simulink model "VDSE_2018b"  (R2018b)
settings: Solver=ode5  StartTime=0.0  StopTime=T_simulation  FixedStep=simulation_step_time  RelTol=1e-3
values from neighbouring files (symbols this model uses):
  A = 2    [vehicle_parameters_script.m]
  bump_height = 0    [vehicle_parameters_script.m]
  bump_length = 1    [vehicle_parameters_script.m]
  bump_time = 1    [vehicle_parameters_script.m]
  Bxf = 17.156    [BCD_Parameters.m]
  Bxr = 17.156    [BCD_Parameters.m]
  Byf = 12.71    [BCD_Parameters.m]
  Byr = 12.71    [BCD_Parameters.m]
  cd = 0.35    [vehicle_parameters_script.m]
  central_diff = 1    [vehicle_parameters_script.m]
  cF = 5000    [vehicle_parameters_script.m]
  clF = -0.15    [vehicle_parameters_script.m]
  clR = -0.20    (= -0.2)    [vehicle_parameters_script.m]
  cp_FA = 30    [vehicle_parameters_script.m]
  cp_RA = 13    [vehicle_parameters_script.m]
  cR = 5000    [vehicle_parameters_script.m]
  ctF = tireF.VERTICAL_DAMPING    [vehicle_parameters_script.m]
  ctR = tireR.VERTICAL_DAMPING    [vehicle_parameters_script.m]
  Cxf = 1.406    [BCD_Parameters.m]
  Cxr = 1.406    [BCD_Parameters.m]
  Cyf = 1.63    [BCD_Parameters.m]
  Cyr = 1.63    [BCD_Parameters.m]
  Dxf = 1.2    [BCD_Parameters.m]
  Dxr = 1.2    [BCD_Parameters.m]
  Dyf = 1.1    [BCD_Parameters.m]
  Dyr = 1.8    [BCD_Parameters.m]
  enableDriverControl = 0    [vehicle_parameters_script.m]
  enableLongDynamics = 1    [vehicle_parameters_script.m]
  enablePowertrain = 1    [vehicle_parameters_script.m]
  front_dr = 3.8    [vehicle_parameters_script.m]
  g = 9.806    [vehicle_parameters_script.m]
  Gear_numbers = [1 2 3 4 5 6]    [vehicle_parameters_script.m]
  GR = [2.9 1.8 1.3 1 0.85 0.75]    [vehicle_parameters_script.m]
  hcog = 0.5    [vehicle_parameters_script.m]
  hpc = 0.0    (= 0)    [vehicle_parameters_script.m]
  hrcF = 0.3    [vehicle_parameters_script.m]
  hrcg = (hrcF*lR+hrcR*lF)/(lF+lR)    (= 0.25108)    [vehicle_parameters_script.m]
  hrcR = 0.2    [vehicle_parameters_script.m]
  huFcog = 0.32    [vehicle_parameters_script.m]
  huRcog = 0.32    [vehicle_parameters_script.m]
  initial_gear = 1    [vehicle_parameters_script.m]
  JwF = 2.45    [vehicle_parameters_script.m]
  JwR = 2.45    [vehicle_parameters_script.m]
  Jx = 430    [vehicle_parameters_script.m]
  Jy = 1309    [vehicle_parameters_script.m]
  Jz = 1461    [vehicle_parameters_script.m]
  kF = 40000    [vehicle_parameters_script.m]
  kR = 35000    [vehicle_parameters_script.m]
  kRF = 0    [vehicle_parameters_script.m]
  kRR = 0    [vehicle_parameters_script.m]
  ktF = tireF.VERTICAL_STIFFNESS    [vehicle_parameters_script.m]
  ktR = tireR.VERTICAL_STIFFNESS    [vehicle_parameters_script.m]
  lF = 1.223    [vehicle_parameters_script.m]
  lR = l-lF    (= 1.277)    [vehicle_parameters_script.m]
  m = 1310    [vehicle_parameters_script.m]
  max_pressure = 1000    [vehicle_parameters_script.m]
  maxrpm = 4000    [vehicle_parameters_script.m]
  mF = 45    [vehicle_parameters_script.m]
  minrpm = 1500    [vehicle_parameters_script.m]
  mR = 50    [vehicle_parameters_script.m]
  output_samping_time = 0.001    [vehicle_parameters_script.m]
  phi0 = 0    [vehicle_parameters_script.m]
  phi_dot0 = 0    [vehicle_parameters_script.m]
  psi0 = 0    [vehicle_parameters_script.m]
  psi_dot0 = 0    [vehicle_parameters_script.m]
  rear_dr = 3.8    [vehicle_parameters_script.m]
  requested_speed = 100/3.6    (= 27.7777777778)    [vehicle_parameters_script.m]
  rF = tireF.UNLOADED_RADIUS    [vehicle_parameters_script.m]
  rho = 1.2    [vehicle_parameters_script.m]
  RPMME = Engine(:,1)    [vehicle_parameters_script.m]
  rR = tireR.UNLOADED_RADIUS    [vehicle_parameters_script.m]
  steer_ratio = 13.25    [vehicle_parameters_script.m]
  TFL = 0    [vehicle_parameters_script.m]
  TFR = 0    [vehicle_parameters_script.m]
  theta0 = 0    [vehicle_parameters_script.m]
  theta_dot0 = 0    [vehicle_parameters_script.m]
  TorqueME = []    [vehicle_parameters_script.m]
  TRL = 0    [vehicle_parameters_script.m]
  TRR = 0    [vehicle_parameters_script.m]
  Vx0 = 100/3.6    (= 27.7777777778)    [vehicle_parameters_script.m]
  Vy0 = 0    [vehicle_parameters_script.m]
  Vz0 = 0    [vehicle_parameters_script.m]
  wF = 1.578    [vehicle_parameters_script.m]
  wR = 1.544    [vehicle_parameters_script.m]
  x0 = 0    [vehicle_parameters_script.m]
  xcog_overall = (2*mR*xR+2*xF*mF+m*xs)/(m+2*mF+2*mR)    (= 1.23475333333)    [vehicle_parameters_script.m]
  y0 = 0    [vehicle_parameters_script.m]
  z0 = 0    [vehicle_parameters_script.m]
  zFL0 = 0    [vehicle_parameters_script.m]
  zFL_dot0 = 0    [vehicle_parameters_script.m]
  zFR0 = 0    [vehicle_parameters_script.m]
  zFR_dot0 = 0    [vehicle_parameters_script.m]
  zRL0 = 0    [vehicle_parameters_script.m]
  zRL_dot0 = 0    [vehicle_parameters_script.m]
  zRR0 = 0    [vehicle_parameters_script.m]
  zRR_dot0 = 0    [vehicle_parameters_script.m]
undefined symbols (not defined in the file or in its folder): exf, exr, eyf, eyr, FNOMINf, FNOMINr, PCX1f, PCX1r, PCY1f, PCY1r, PDX1f, PDX1r, PDX2f, PDX2r, PDY1f, PDY1r, PDY2f, PDY2r, PDY3f, PDY3r, PEX1f, PEX1r, PEX2f, PEX2r, PEX3f, PEX3r, PEX4f, PEX4r, PEY1f, PEY1r, PEY2f, PEY2r, PEY3f, PEY3r, PEY4f, PEY4r, PHX1f, PHX1r, PHX2f, PHX2r, PHY1f, PHY1r, PHY2f, PHY2r, PHY3f, PHY3r, PKX1f, PKX1r, PKX2f, PKX2r, PKX3f, PKX3r, PKY1f, PKY1r, PKY2f, PKY2r, PKY3f, PKY3r, PVX1f, PVX1r ... (+122)
libraries: simulink x7, mfeval_LIB x4
(part 1 of 6)
settings Model: Creator=Christos  LastModifiedBy=Christos

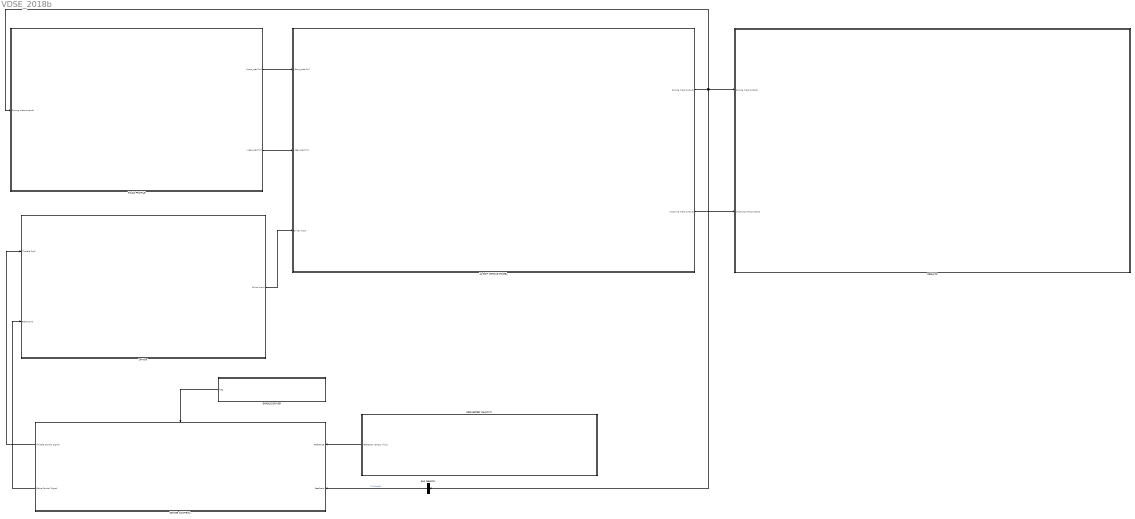
== system VDSE_2018b ==
  14-DOF VEHICLE MODEL : Subsystem
  Bus Selector : BusSelector  OutputSignals=Longitudinal Dynamics.Vx [m/s]
  DRIVER : Subsystem
  DRIVER CONTROL : Subsystem  TreatAsAtomicUnit=on
  "ENABLE DRIVER " : Subsystem
  REQUESTED VELOCITY : Subsystem
  RESULTS : Subsystem
  ROAD PROFILE : Subsystem
  wires:
  14-DOF VEHICLE MODEL/2(Unsprung mass outputs) -> RESULTS/2(Unsprung mass outputs)
  ROAD PROFILE/2(yrear_road [m]) -> 14-DOF VEHICLE MODEL/2(yrear_road [m])
  Bus Selector/1 -> DRIVER CONTROL/2(Feedback)  "<Vx [m/s]>"
  ROAD PROFILE/1(yfront_road [m]) -> 14-DOF VEHICLE MODEL/1(yfront_road [m])
  DRIVER/1(Driver Input) -> 14-DOF VEHICLE MODEL/3(Driver Input)
  DRIVER CONTROL/2(Brake Control Signal) -> DRIVER/2(Brake Cmd)
  14-DOF VEHICLE MODEL/1(Sprung mass outputs) -> Bus Selector/1, RESULTS/1(Sprung mass outputs), ROAD PROFILE/1(Sprung mass outputs)
  DRIVER CONTROL/1(Throttle Control Signal) -> DRIVER/1(Throttle Cmd)
  REQUESTED VELOCITY/1(reference velocity [m/s]) -> DRIVER CONTROL/1(Reference)
  "ENABLE DRIVER "/1(flag) -> DRIVER CONTROL/Enable

== system VDSE_2018b/14-DOF VEHICLE MODEL ==
  yfront_road [m] : Inport
  yrear_road [m] : Inport  Port=2
  Driver Input : Inport  Port=3
  Driver Input1 : InportShadow  Port=3
  EQUATIONS OF MOTION FOR CHASSIS : Subsystem
  POWERTRAIN AND BRAKES : Subsystem
  SUSPENSION : Subsystem
  WHEEL ASSEMBLY : Subsystem  Variant=on
  Sprung mass outputs : Outport
  Unsprung mass outputs : Outport  Port=2
  wires:
  EQUATIONS OF MOTION FOR CHASSIS/1(Sprung mass outputs) -> Sprung mass outputs/1, SUSPENSION/3(sprung mass outputs), WHEEL ASSEMBLY/2(sprung mass outputs)  "Sprung mass outputs"
  yfront_road [m]/1 -> SUSPENSION/1(yfront_road [m])
  yrear_road [m]/1 -> SUSPENSION/2(yrear_road [m])
  WHEEL ASSEMBLY/1(Tyre Forces and Moments) -> EQUATIONS OF MOTION FOR CHASSIS/2(Tyre Forces and Moments)
  SUSPENSION/1(" Unsprung masses output") -> WHEEL ASSEMBLY/3(unsprung masses outputs), EQUATIONS OF MOTION FOR CHASSIS/3(unsprung masses outputs), Unsprung mass outputs/1  "unsprung masses outputs"
  Driver Input/1 -> EQUATIONS OF MOTION FOR CHASSIS/1(Steer Input [rad]), WHEEL ASSEMBLY/1(steer input [rad])
  WHEEL ASSEMBLY/2(Wheel Speeds [rad/s]) -> POWERTRAIN AND BRAKES/1(Wheels speed [rad/s])
  Driver Input1/1 -> POWERTRAIN AND BRAKES/2(Driver)
  POWERTRAIN AND BRAKES/1(Torques [Nm]) -> [Torques]
  [Torques] -> WHEEL ASSEMBLY/4(Torques [Nm])

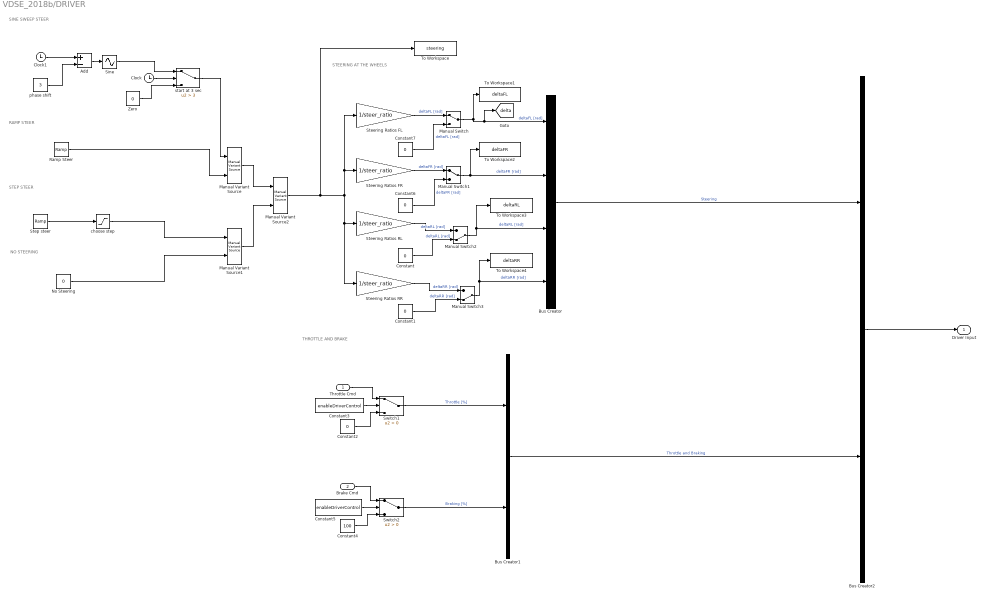
== system VDSE_2018b/DRIVER ==
  note: THROTTLE AND BRAKE
  note: STEERING AT THE WHEELS
  note: NO STEERING
  note: STEP STEER
  note: RAMP STEER
  note: SINE SWEEP STEER
  Throttle Cmd : Inport
  Brake Cmd : Inport  Port=2
  Add : Sum  Inputs=+-
  Bus Creator : BusCreator  Inputs=4
  Bus Creator1 : BusCreator  Inputs=2
  Bus Creator2 : BusCreator  Inputs=2
  Clock : Clock
  Clock1 : Clock
  Constant{,1..2,6..7} (5 alike) : Constant  Value=0
  Constant3 : Constant  Value=enableDriverControl
  Constant4 : Constant  Value=100
  Constant5 : Constant  Value=enableDriverControl
  Manual Variant Source : simulink/Signal Routing/Manual Variant Source  NumChoices=2  LabelModeActiveChoice=V_2
      settings: SourceProductName=Simulink
  Manual Variant Source1 : simulink/Signal Routing/Manual Variant Source  NumChoices=2  LabelModeActiveChoice=V_2
      settings: SourceProductName=Simulink
  Manual Variant Source2 : simulink/Signal Routing/Manual Variant Source  NumChoices=2  LabelModeActiveChoice=V_1
      settings: SourceProductName=Simulink
  Manual Switch : ManualSwitch
  Manual Switch1 : ManualSwitch
  Manual Switch2 : ManualSwitch  CurrentSetting=0
  Manual Switch3 : ManualSwitch  CurrentSetting=0
  No Steering : Constant  Value=0
  Ramp Steer : simulink/Sources/Ramp  slope=10*pi/180  start=1  InitialOutput=0
  Sine : Sin  TimeSource=Use external signal  Amplitude=30*pi/180  SampleTime=0
  Steering Ratios FL : Gain  Gain=1/steer_ratio
  Steering Ratios FR : Gain  Gain=1/steer_ratio
  Steering Ratios RL : Gain  Gain=1/steer_ratio
  Steering Ratios RR : Gain  Gain=1/steer_ratio
  Step steer : simulink/Sources/Ramp  slope=1400*pi/180  start=15  InitialOutput=0
  Switch1 : Switch  Criteria=u2 > Threshold
  Switch2 : Switch  Criteria=u2 > Threshold
  To Workspace : ToWorkspace  VariableName=steering  SaveFormat=Timeseries  SampleTime=output_samping_time
  To Workspace1 : ToWorkspace  VariableName=deltaFL  SaveFormat=Timeseries  SampleTime=output_samping_time
  To Workspace2 : ToWorkspace  VariableName=deltaFR  SaveFormat=Timeseries  SampleTime=output_samping_time
  To Workspace3 : ToWorkspace  VariableName=deltaRL  SaveFormat=Timeseries  SampleTime=output_samping_time
  To Workspace4 : ToWorkspace  VariableName=deltaRR  SaveFormat=Timeseries  SampleTime=output_samping_time
  Zero : Constant  Value=0  OutDataTypeStr=Inherit: Inherit via back propagation
  "choose step " : Saturate  UpperLimit=700*pi/180  LowerLimit=0
  "phase shift " : Constant  Value=3
  start at 3 sec : Switch  Criteria=u2 > Threshold  Threshold=3
  Driver Input : Outport
  tag scope: delta=global
  wires:
  Zero/1 -> start at 3 sec/3
  Manual Switch3/1 -> To Workspace4/1, Bus Creator/4  "deltaRR [rad]"
  "phase shift "/1 -> Add/2
  Add/1 -> Sine/1
  Clock1/1 -> Add/1
  Clock/1 -> start at 3 sec/2
  start at 3 sec/1 -> Manual Variant Source/1
  "choose step "/1 -> Manual Variant Source1/1
  Manual Variant Source/1 -> Manual Variant Source2/1
  Sine/1 -> start at 3 sec/1
  No Steering/1 -> Manual Variant Source1/2
  Manual Variant Source1/1 -> Manual Variant Source2/2
  Manual Switch/1 -> [delta], Bus Creator/1, To Workspace1/1  "deltaFL [rad]"
  Manual Variant Source2/1 -> To Workspace/1, Steering Ratios FL/1, Steering Ratios FR/1, Steering Ratios RL/1, Steering Ratios RR/1
  Step steer/1 -> "choose step "/1
  Ramp Steer/1 -> Manual Variant Source/2
  Manual Switch2/1 -> To Workspace3/1, Bus Creator/3  "deltaRL [rad]"
  Constant2/1 -> Switch1/3
  Bus Creator2/1 -> Driver Input/1
  Bus Creator/1 -> Bus Creator2/1  "Steering"
  Bus Creator1/1 -> Bus Creator2/2  "Throttle and Braking"
  Throttle Cmd/1 -> Switch1/1
  Constant3/1 -> Switch1/2
  Constant1/1 -> Manual Switch3/2  "deltaRR [rad]"
  Constant/1 -> Manual Switch2/2  "deltaRL [rad]"
  Steering Ratios RL/1 -> Manual Switch2/1  "deltaRL [rad]"
  Steering Ratios FL/1 -> Manual Switch/1  "deltaFL [rad]"
  Manual Switch1/1 -> To Workspace2/1, Bus Creator/2  "deltaFR [rad]"
  Steering Ratios FR/1 -> Manual Switch1/1  "deltaFR [rad]"
  Brake Cmd/1 -> Switch2/1
  Constant5/1 -> Switch2/2
  Constant4/1 -> Switch2/3
  Switch2/1 -> Bus Creator1/2  "Braking [%]"
  Constant6/1 -> Manual Switch1/2  "deltaFR [rad]"
  Constant7/1 -> Manual Switch/2  "deltaFL [rad]"
  Switch1/1 -> Bus Creator1/1  "Throttle [%]"
  Steering Ratios RR/1 -> Manual Switch3/1  "deltaRR [rad]"

== system VDSE_2018b/DRIVER CONTROL ==
  Reference : Inport
  Feedback : Inport  Port=2
  Enable : EnablePort
  Abs : Abs
  Add : Sum  Inputs=+-
  Driver : simulink/Continuous/PID Controller  Controller=PID  Form=Parallel  TimeDomain=Continuous-time  SampleTime=-1  IntegratorMethod=Forward Euler  FilterMethod=Forward Euler  ControllerParametersSource=internal  P=200  I=0  D=50  UseFilter=on  N=10  TunerSelectOption=Transfer Function Based (PID Tuner App)  InitialConditionSource=internal  InitialConditionForIntegrator=0  InitialConditionForFilter=0  DifferentiatorICPrevScaledInput=0  ExternalReset=none  TrackingMode=off  Kt=1  LimitOutput=off  UpperSaturationLimit=inf  LowerSaturationLimit=-inf  LinearizeAsGain=on  AntiWindupMode=none  Kb=1  POutMin=[]  POutMax=[]  IOutMin=[]  IOutMax=[]  DOutMin=[]  DOutMax=[]  NOutMin=[]  NOutMax=[]  SumOutMin=[]  SumOutMax=[]  SaturationOutMin=[]  SaturationOutMax=[]  PParamMin=[]  PParamMax=[]  IParamMin=[]  IParamMax=[]  DParamMin=[]  DParamMax=[]  NParamMin=[]  NParamMax=[]  KbParamMin=[]  KbParamMax=[]  KtParamMin=[]  KtParamMax=[]  KbOutMin=[]  KbOutMax=[]  KtOutMin=[]  KtOutMax=[]  IntegratorOutMin=[]  IntegratorOutMax=[]  FilterOutMin=[]  FilterOutMax=[]  SumI1OutMin=[]  SumI1OutMax=[]  SumI2OutMin=[]  SumI2OutMax=[]  SumI3OutMin=[]  SumI3OutMax=[]  SumI4OutMin=[]  SumI4OutMax=[]  SumDOutMin=[]  SumDOutMax=[]  DifferentiatorOutMin=[]  DifferentiatorOutMax=[]  FilterDiffOutCoefMin=[]  FilterDiffOutCoefMax=[]  ReciprocalOutMin=[]  ReciprocalOutMax=[]  SumDenOutMin=[]  SumDenOutMax=[]  SumNumOutMin=[]  SumNumOutMax=[]  DivideOutMin=[]  DivideOutMax=[]  IntegratorContinuousStateAttributes=''  IntegratorStateMustResolveToSignalObject=off  IntegratorRTWStateStorageClass=Auto  FilterContinuousStateAttributes=''  FilterStateMustResolveToSignalObject=off  FilterRTWStateStorageClass=Auto  ParallelPVariant=InternalParameters  IdealPVariant=Disabled  IVariant=InternalParameters  DVariant=InternalParameters  IntegratorVariant=Continuous  SatVariant=Disabled  AWVariant=Passthrough  PCopyVariant=Disabled  TRVariant=Disabled  FdbkBlocksVariant=Forward  IdealPFdbkVariant=Disabled  SatFdbkVariant=Disabled  DerivativeFilterVariant=ContFilter  NVariant=InternalParameters  NCopyVariant=Disabled  FilterICVariant=InternalICsFilter  IntegratorICVariant=InternalICs  ExternalResetVariant=Disabled  TRSumVariant=Passthrough  SumFdbkVariant=Disabled  SumVariant=Sum_PID
  MATLAB Function : MATLAB Function  TreatAsAtomicUnit=on
  Saturation : Saturate  UpperLimit=100  LowerLimit=0
  Saturation1 : Saturate  UpperLimit=0  LowerLimit=-100
  Scope : Scope  NumInputPorts=2
  Scope1 : Scope
  Throttle Control Signal : Outport
  Brake Control Signal : Outport  Port=2
  wires:
  Reference/1 -> Add/1
  Add/1 -> Scope1/1, Driver/1  "Error"
  Driver/1 -> Saturation/1, Saturation1/1
  Saturation/1 -> Scope/1, Throttle Control Signal/1  "Throttle Command [%]"
  Saturation1/1 -> Scope/2, MATLAB Function/1(brake)  "Brake Command [%]"
  MATLAB Function/1(Brake_Cmd) -> Abs/1
  Feedback/1 -> MATLAB Function/2(Vx), Add/2
  Abs/1 -> Brake Control Signal/1

== system VDSE_2018b/ENABLE DRIVER  ==
  Constant1 : Constant  Value=enableDriverControl
  flag : Outport
  wires:
  Constant1/1 -> flag/1

== system VDSE_2018b/REQUESTED VELOCITY ==
  note: REQUESTED VELOCITY
  Constant : Constant  Value=requested_speed
  Manual Switch : ManualSwitch
  Sine Wave : Sin  Amplitude=10/3.6  Bias=90/3.6  Frequency=0.1  SampleTime=0
  reference velocity [m/s] : Outport
  tag scope: ref_vel=global
  wires:
  Manual Switch/1 -> reference velocity [m/s]/1, [ref_vel]  "reference velocity [m/s]"
  Sine Wave/1 -> Manual Switch/2
  Constant/1 -> Manual Switch/1

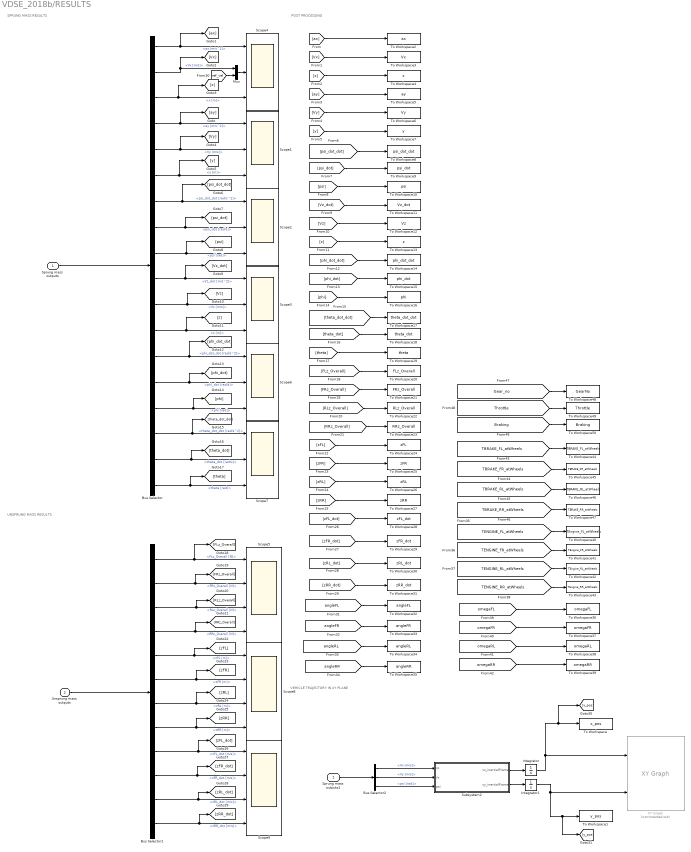
== system VDSE_2018b/RESULTS ==
  note: POST PROCESSING
  note: VEHICLE TRAJECTORY IN XY PLANE
  note: UNSPRUNG MASS RESULTS
  note: SPRUNG MASS RESULTS
  Sprung mass outputs : Inport
  Unsprung mass outputs : Inport  Port=2
  Bus Selector : BusSelector  OutputSignals=Longitudinal Dynamics.ax [m/s^2],Longitudinal Dynamics.Vx [m/s],Longitudinal Dynamics.x [m],Lateral Dynamics.ay [m/s^2],Lateral Dynamics.Vy [m/s],Lateral Dynamics.y [m],Yaw dynamics.psi_dot_dot [rad/s^2],Yaw dynamics.psi_dot [rad/s],Yaw dynamics.psi [rad],Vertical Dynamics.Vz_dot [m/s^2],Vertical Dynamics.Vz [m/s],Vertical Dynamics.z [m],Roll Dynamics.phi_dot_dot [rad/s^2],Roll Dynamics.phi_dot [rad/s],Roll Dynamics.phi [rad],Pitch Dynamics.theta_dot_dot [rad/s^2],Pitch Dynamics.theta_dot [rad/s],Pitch Dynamics.theta [rad]
  Bus Selector1 : BusSelector  OutputSignals=Unsprung masses z Forces [N].FLz_Overall [N],Unsprung masses z Forces [N].FRz_Overall [N],Unsprung masses z Forces [N].RLz_Overall [N],Unsprung masses z Forces [N].RRz_Overall [N],Unsprung masses z displacement [m].zFL [m],Unsprung masses z displacement [m].zFR [m],Unsprung masses z displacement [m].zRL [m],Unsprung masses z displacement [m].zRR [m],Unsprung masses z Velocities [m/s].zFL_dot [m/s],Unsprung masses z Velocities [m/s].zFR_dot [m/s],Unsprung masses z Velocities [m/s].zRL_dot [m/s],Unsprung masses z Velocities [m/s].zRR_dot [m/s]
  Bus Selector2 : BusSelector  OutputSignals=Longitudinal Dynamics.Vx [m/s],Lateral Dynamics.Vy [m/s],Yaw dynamics.psi [rad]
  Integrator : Integrator
  Integrator1 : Integrator
  Mux : Mux  Inputs=2
  Scope{1..4,6..7} (6 alike) : Scope  NumInputPorts=3
  Scope5 : Scope  NumInputPorts=4
  Scope8 : Scope  NumInputPorts=4
  Scope9 : Scope  NumInputPorts=4
  Sprung mass outputs1 : InportShadow
  Subsystem2 : Subsystem
  To Workspace : ToWorkspace  VariableName=x_pos  SaveFormat=Timeseries  SampleTime=output_samping_time
  To Workspace1 : ToWorkspace  VariableName=y_pos  SaveFormat=Timeseries  SampleTime=output_samping_time
  To Workspace10 : ToWorkspace  VariableName=psi  SaveFormat=Timeseries  SampleTime=output_samping_time
  To Workspace11 : ToWorkspace  VariableName=Vz_dot  SaveFormat=Timeseries  SampleTime=output_samping_time
  To Workspace12 : ToWorkspace  VariableName=Vz  SaveFormat=Timeseries  SampleTime=output_samping_time
  To Workspace13 : ToWorkspace  VariableName=z  SaveFormat=Timeseries  SampleTime=output_samping_time
  To Workspace14 : ToWorkspace  VariableName=phi_dot_dot  SaveFormat=Timeseries  SampleTime=output_samping_time
  To Workspace15 : ToWorkspace  VariableName=phi_dot  SaveFormat=Timeseries  SampleTime=output_samping_time
  To Workspace16 : ToWorkspace  VariableName=phi  SaveFormat=Timeseries  SampleTime=output_samping_time
  To Workspace17 : ToWorkspace  VariableName=theta_dot_dot  SaveFormat=Timeseries  SampleTime=output_samping_time
  To Workspace18 : ToWorkspace  VariableName=theta_dot  SaveFormat=Timeseries  SampleTime=output_samping_time
  To Workspace19 : ToWorkspace  VariableName=theta  SaveFormat=Timeseries  SampleTime=output_samping_time
  To Workspace2 : ToWorkspace  VariableName=ax  SaveFormat=Timeseries  SampleTime=output_samping_time
  To Workspace20 : ToWorkspace  VariableName=FLz_Overall  SaveFormat=Timeseries  SampleTime=output_samping_time
  To Workspace21 : ToWorkspace  VariableName=FRz_Overall  SaveFormat=Timeseries  SampleTime=output_samping_time
  To Workspace22 : ToWorkspace  VariableName=RLz_Overall  SaveFormat=Timeseries  SampleTime=output_samping_time
  To Workspace23 : ToWorkspace  VariableName=RRz_Overall  SaveFormat=Timeseries  SampleTime=output_samping_time
  To Workspace24 : ToWorkspace  VariableName=zFL  SaveFormat=Timeseries  SampleTime=output_samping_time
  To Workspace25 : ToWorkspace  VariableName=zFR  SaveFormat=Timeseries  SampleTime=output_samping_time
  To Workspace26 : ToWorkspace  VariableName=zRL  SaveFormat=Timeseries  SampleTime=output_samping_time
  To Workspace27 : ToWorkspace  VariableName=zRR  SaveFormat=Timeseries  SampleTime=output_samping_time
  To Workspace28 : ToWorkspace  VariableName=zFL_dot  SaveFormat=Timeseries  SampleTime=output_samping_time
  To Workspace29 : ToWorkspace  VariableName=zFR_dot  SaveFormat=Timeseries  SampleTime=output_samping_time
  To Workspace3 : ToWorkspace  VariableName=Vx  SaveFormat=Timeseries  SampleTime=output_samping_time
  To Workspace30 : ToWorkspace  VariableName=zRL_dot  SaveFormat=Timeseries  SampleTime=output_samping_time
  To Workspace31 : ToWorkspace  VariableName=zRR_dot  SaveFormat=Timeseries  SampleTime=output_samping_time
  To Workspace32 : ToWorkspace  VariableName=angleFL  SaveFormat=Timeseries  SampleTime=output_samping_time
  To Workspace33 : ToWorkspace  VariableName=angleFR  SaveFormat=Timeseries  SampleTime=output_samping_time
  To Workspace34 : ToWorkspace  VariableName=angleRL  SaveFormat=Timeseries  SampleTime=output_samping_time
  To Workspace35 : ToWorkspace  VariableName=angleRR  SaveFormat=Timeseries  SampleTime=output_samping_time
  To Workspace36 : ToWorkspace  VariableName=omegaFL  SaveFormat=Timeseries  SampleTime=output_samping_time
  To Workspace37 : ToWorkspace  VariableName=omegaFR  SaveFormat=Timeseries  SampleTime=output_samping_time
  To Workspace38 : ToWorkspace  VariableName=omegaRL  SaveFormat=Timeseries  SampleTime=output_samping_time
  To Workspace39 : ToWorkspace  VariableName=omegaRR  SaveFormat=Timeseries  SampleTime=output_samping_time
  To Workspace4 : ToWorkspace  VariableName=x  SaveFormat=Timeseries  SampleTime=output_samping_time
  To Workspace40 : ToWorkspace  VariableName=TEngine_FL_atWheels  SaveFormat=Timeseries  SampleTime=output_samping_time
  To Workspace41 : ToWorkspace  VariableName=TEngine_FR_atWheels  SaveFormat=Timeseries  SampleTime=output_samping_time
  To Workspace42 : ToWorkspace  VariableName=TEngine_RL_atWheels  SaveFormat=Timeseries  SampleTime=output_samping_time
  To Workspace43 : ToWorkspace  VariableName=TEngine_RR_atWheels  SaveFormat=Timeseries  SampleTime=output_samping_time
  To Workspace44 : ToWorkspace  VariableName=TBRAKE_FL_atWheels  SaveFormat=Timeseries  SampleTime=output_samping_time
  To Workspace45 : ToWorkspace  VariableName=TBRAKE_FR_atWheels  SaveFormat=Timeseries  SampleTime=output_samping_time
  To Workspace46 : ToWorkspace  VariableName=TBRAKE_RL_atWheels  SaveFormat=Timeseries  SampleTime=output_samping_time
  To Workspace47 : ToWorkspace  VariableName=TBRAKE_RR_atWheels  SaveFormat=Timeseries  SampleTime=output_samping_time
  To Workspace48 : ToWorkspace  VariableName=GearNo  SaveFormat=Timeseries  SampleTime=output_samping_time
  To Workspace49 : ToWorkspace  VariableName=Throttle  SaveFormat=Timeseries  SampleTime=output_samping_time
  To Workspace5 : ToWorkspace  VariableName=ay  SaveFormat=Timeseries  SampleTime=output_samping_time
  To Workspace50 : ToWorkspace  VariableName=Braking  SaveFormat=Timeseries  SampleTime=output_samping_time
  To Workspace6 : ToWorkspace  VariableName=Vy  SaveFormat=Timeseries  SampleTime=output_samping_time
  To Workspace7 : ToWorkspace  VariableName=y  SaveFormat=Timeseries  SampleTime=output_samping_time
  To Workspace8 : ToWorkspace  VariableName=psi_dot_dot  SaveFormat=Timeseries  SampleTime=output_samping_time
  To Workspace9 : ToWorkspace  VariableName=psi_dot  SaveFormat=Timeseries  SampleTime=output_samping_time
  XY Graph : simulink/Sinks/XY Graph  Commented=on  xmin=-2500  xmax=1500  ymin=-2500  ymax=1500  st=-1
  wires:
  Integrator1/1 -> [y_pos], To Workspace1/1, XY Graph/2
  Integrator/1 -> [x_pos], To Workspace/1, XY Graph/1
  Subsystem2/1(vx_inertialFrame) -> Integrator/1
  Subsystem2/2(vy_inertialFrame) -> Integrator1/1
  Sprung mass outputs/1 -> Bus Selector/1
  Unsprung mass outputs/1 -> Bus Selector1/1
  Bus Selector/1 -> [ax], Scope4/1  "<ax [m/s^2]>"
  Bus Selector/2 -> Mux/1, [Vx]  "<Vx [m/s]>"
  Bus Selector/3 -> [x], Scope4/3  "<x [m]>"
  Bus Selector/4 -> [ay], Scope1/1  "<ay [m/s^2]>"
  Bus Selector/5 -> [Vy], Scope1/2  "<Vy [m/s]>"
  Bus Selector/6 -> [y], Scope1/3  "<y [m]>"
  Bus Selector/7 -> [psi_dot_dot], Scope2/1  "<psi_dot_dot [rad/s^2]>"
  Bus Selector/8 -> [psi_dot], Scope2/2  "<psi_dot [rad/s]>"
  Bus Selector/9 -> [psi], Scope2/3  "<psi [rad]>"
  Bus Selector/10 -> [Vz_dot], Scope3/1  "<Vz_dot [m/s^2]>"
  Bus Selector/11 -> [Vz], Scope3/2  "<Vz [m/s]>"
  Bus Selector/12 -> [z], Scope3/3  "<z [m]>"
  Bus Selector/13 -> [phi_dot_dot], Scope6/1  "<phi_dot_dot [rad/s^2]>"
  Bus Selector/14 -> [phi_dot], Scope6/2  "<phi_dot [rad/s]>"
  Bus Selector/15 -> [phi], Scope6/3  "<phi [rad]>"
  Bus Selector/16 -> [theta_dot_dot], Scope7/1  "<theta_dot_dot [rad/s^2]>"
  Bus Selector/17 -> [theta_dot], Scope7/2  "<theta_dot [rad/s]>"
  Bus Selector/18 -> [theta], Scope7/3  "<theta [rad]>"
  Bus Selector1/1 -> [FLz_Overall], Scope5/1  "<FLz_Overall [N]>"
  Bus Selector1/2 -> [FRz_Overall], Scope5/2  "<FRz_Overall [N]>"
  Bus Selector1/3 -> [RLz_Overall], Scope5/3  "<RLz_Overall [N]>"
  Bus Selector1/4 -> [RRz_Overall], Scope5/4  "<RRz_Overall [N]>"
  Bus Selector1/5 -> [zFL], Scope8/1  "<zFL [m]>"
  Bus Selector1/6 -> [zFR], Scope8/2  "<zFR [m]>"
  Bus Selector1/7 -> [zRL], Scope8/3  "<zRL [m]>"
  Bus Selector1/8 -> [zRR], Scope8/4  "<zRR [m]>"
  Bus Selector1/9 -> [zFL_dot], Scope9/1  "<zFL_dot [m/s]>"
  Bus Selector1/10 -> [zFR_dot], Scope9/2  "<zFR_dot [m/s]>"
  Bus Selector1/11 -> [zRL_dot], Scope9/3  "<zRL_dot [m/s]>"
  Bus Selector1/12 -> [zRR_dot], Scope9/4  "<zRR_dot [m/s]>"
  Sprung mass outputs1/1 -> Bus Selector2/1
  Bus Selector2/1 -> Subsystem2/1(vx)  "<Vx [m/s]>"
  Bus Selector2/2 -> Subsystem2/2(vy)  "<Vy [m/s]>"
  Bus Selector2/3 -> Subsystem2/3(psi)  "<psi [rad]>"
  [ax] -> To Workspace2/1
  [Vx] -> To Workspace3/1
  [x] -> To Workspace4/1
  [ay] -> To Workspace5/1
  [Vy] -> To Workspace6/1
  [y] -> To Workspace7/1
  [psi_dot_dot] -> To Workspace8/1
  [psi_dot] -> To Workspace9/1
  [psi] -> To Workspace10/1
  [Vz_dot] -> To Workspace11/1
  [Vz] -> To Workspace12/1
  [z] -> To Workspace13/1
  [phi_dot_dot] -> To Workspace14/1
  [phi_dot] -> To Workspace15/1
  [phi] -> To Workspace16/1
  [theta_dot_dot] -> To Workspace17/1
  [theta_dot] -> To Workspace18/1
  [theta] -> To Workspace19/1
  [FLz_Overall] -> To Workspace20/1
  [FRz_Overall] -> To Workspace21/1
  [RLz_Overall] -> To Workspace22/1
  [RRz_Overall] -> To Workspace23/1
  [zFL] -> To Workspace24/1
  [zFR] -> To Workspace25/1
  [zRL] -> To Workspace26/1
  [zRR] -> To Workspace27/1
  [zFL_dot] -> To Workspace28/1
  [zFR_dot] -> To Workspace29/1
  [zRL_dot] -> To Workspace30/1
  [zRR_dot] -> To Workspace31/1
  Mux/1 -> Scope4/2
  [ref_vel] -> Mux/2
  [angleFL] -> To Workspace32/1
  [angleFR] -> To Workspace33/1
  [angleRL] -> To Workspace34/1
  [angleRR] -> To Workspace35/1
  [omegaFL] -> To Workspace36/1
  [omegaFR] -> To Workspace37/1
  [omegaRL] -> To Workspace38/1
  [omegaRR] -> To Workspace39/1
  [TENGINE_FL_atWheels] -> To Workspace40/1
  [TENGINE_FR_atWheels] -> To Workspace41/1
  [TENGINE_RL_atWheels] -> To Workspace42/1
  [TENGINE_RR_atWheels] -> To Workspace43/1
  [TBRAKE_FL_atWheels] -> To Workspace44/1
  [TBRAKE_FR_atWheels] -> To Workspace45/1
  [TBRAKE_RL_atWheels] -> To Workspace46/1
  [TBRAKE_RR_atWheels] -> To Workspace47/1
  [Gear_no] -> To Workspace48/1
  [Throttle] -> To Workspace49/1
  [Braking] -> To Workspace50/1

== system VDSE_2018b/ROAD PROFILE ==
  note: GENERATION OF ROAD PROFILE
  Sprung mass outputs : Inport
  Bus Creator : BusCreator  Inputs=2
  Bus Creator1 : BusCreator  Inputs=2
  Bus Selector : BusSelector  OutputSignals=Longitudinal Dynamics.Vx [m/s]
  Clock : Clock
  Constant : Constant  Value=bump_height
  Constant1 : Constant  Value=bump_length
  Constant2 : Constant  Value=bump_time
  Constant3 : Constant  Value=lF
  Constant4 : Constant  Value=lR
  GENERATION OF ROAD PROFILE : MATLAB Function  TreatAsAtomicUnit=on
  yfront_road [m] : Outport
  yrear_road [m] : Outport  Port=2
  wires:
  Clock/1 -> GENERATION OF ROAD PROFILE/1(sim_time)  "Simulation's clock"
  Constant/1 -> GENERATION OF ROAD PROFILE/2(bump_height)  "Height of the bump"
  Constant1/1 -> GENERATION OF ROAD PROFILE/3(bump_length)  "Length of the bump"
  Constant2/1 -> GENERATION OF ROAD PROFILE/6(bump_time)  "Start time of the bump"
  GENERATION OF ROAD PROFILE/1(yFL_road) -> Bus Creator/1  "yFL_road [m]"
  GENERATION OF ROAD PROFILE/2(yFR_road) -> Bus Creator/2  "yFR_road [m]"
  Constant4/1 -> GENERATION OF ROAD PROFILE/5(lR)  "Rear vehicle's wheelbase"
  Constant3/1 -> GENERATION OF ROAD PROFILE/4(lF)  "Front vehicle's wheelbase"
  Sprung mass outputs/1 -> Bus Selector/1
  Bus Selector/1 -> GENERATION OF ROAD PROFILE/7(Vx)  "<Vx [m/s]>"
  Bus Creator/1 -> yfront_road [m]/1
  Bus Creator1/1 -> yrear_road [m]/1
  GENERATION OF ROAD PROFILE/3(yRL_road) -> Bus Creator1/1  "yRL_road [m]"
  GENERATION OF ROAD PROFILE/4(yRR_road) -> Bus Creator1/2  "yRR_road [m]"

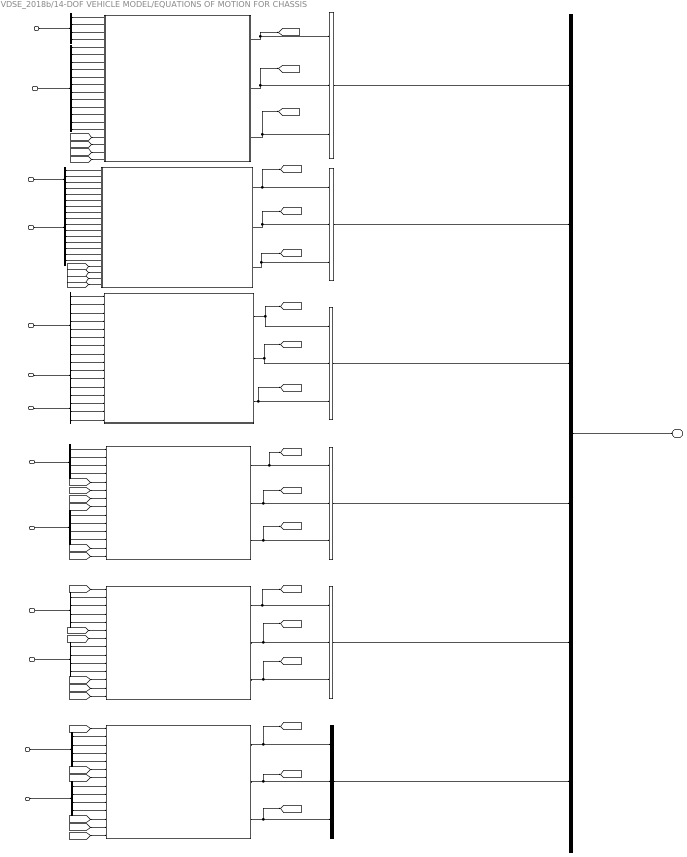
== system VDSE_2018b/14-DOF VEHICLE MODEL/EQUATIONS OF MOTION FOR CHASSIS ==
  note: RIDE
  note: HANDLING
  Steer Input [rad] : Inport
  Tyre Forces and Moments : Inport  Port=2
  unsprung masses outputs : Inport  Port=3
  Bus Creator : BusCreator  Inputs=6
  Bus Creator{1..6} (6 alike) : BusCreator  Inputs=3
  Bus Selector : BusSelector  OutputSignals=Unsprung masses z displacement [m].zFL [m],Unsprung masses z displacement [m].zFR [m],Unsprung masses z displacement [m].zRR [m],Unsprung masses z displacement [m].zRL [m]
  Bus Selector1 : BusSelector  OutputSignals=Unsprung masses z Velocities [m/s].zFL_dot [m/s],Unsprung masses z Velocities [m/s].zFR_dot [m/s],Unsprung masses z Velocities [m/s].zRR_dot [m/s],Unsprung masses z Velocities [m/s].zRL_dot [m/s]
  Bus Selector10 : BusSelector  OutputSignals=Tyre y Forces [N].fFLy [N],Tyre y Forces [N].fFRy [N],Tyre y Forces [N].fRLy [N],Tyre y Forces [N].fRRy [N],Tyre x Forces [N].fFLx [N],Tyre x Forces [N].fFRx [N],Tyre x Forces [N].fRLx [N],Tyre x Forces [N].fRRx [N]
  Bus Selector12 : BusSelector  OutputSignals=Steering.deltaFL [rad],Steering.deltaFR [rad],Steering.deltaRL [rad],Steering.deltaRR [rad]
  Bus Selector13 : BusSelector  OutputSignals=Steering.deltaFL [rad],Steering.deltaFR [rad],Steering.deltaRL [rad],Steering.deltaRR [rad]
  Bus Selector14 : BusSelector  OutputSignals=Steering.deltaFL [rad],Steering.deltaFR [rad],Steering.deltaRL [rad],Steering.deltaRR [rad]
  Bus Selector2 : BusSelector  OutputSignals=Unsprung masses z displacement [m].zFL [m],Unsprung masses z displacement [m].zFR [m],Unsprung masses z displacement [m].zRR [m],Unsprung masses z displacement [m].zRL [m]
  Bus Selector3 : BusSelector  OutputSignals=Unsprung masses z Velocities [m/s].zFL_dot [m/s],Unsprung masses z Velocities [m/s].zFR_dot [m/s],Unsprung masses z Velocities [m/s].zRR_dot [m/s],Unsprung masses z Velocities [m/s].zRL_dot [m/s]
  Bus Selector4 : BusSelector  OutputSignals=Unsprung masses z displacement [m].zFL [m],Unsprung masses z displacement [m].zFR [m],Unsprung masses z displacement [m].zRR [m],Unsprung masses z displacement [m].zRL [m]
  Bus Selector5 : BusSelector  OutputSignals=Unsprung masses z Velocities [m/s].zFL_dot [m/s],Unsprung masses z Velocities [m/s].zFR_dot [m/s],Unsprung masses z Velocities [m/s].zRR_dot [m/s],Unsprung masses z Velocities [m/s].zRL_dot [m/s]
  Bus Selector6 : BusSelector  OutputSignals=Tyre x Forces [N].fFLx [N],Tyre x Forces [N].fFRx [N],Tyre x Forces [N].fRLx [N],Tyre x Forces [N].fRRx [N],Tyre y Forces [N].fFLy [N],Tyre y Forces [N].fFRy [N],Tyre y Forces [N].fRLy [N],Tyre y Forces [N].fRRy [N],Tyre My Moments [Nm].mFLy [Nm],Tyre My Moments [Nm].mFRy [Nm],Tyre My Moments [Nm].mRLy [Nm],Tyre My Moments [Nm].mRRy [Nm]
  Bus Selector7 : BusSelector  OutputSignals=Tyre Mz Moments [Nm].mFLz [Nm],Tyre Mz Moments [Nm].mFRz [Nm],Tyre Mz Moments [Nm].mRLz [Nm],Tyre Mz Moments [Nm].mRRz [Nm]
  Bus Selector8 : BusSelector  OutputSignals=Tyre x Forces [N].fFLx [N],Tyre x Forces [N].fFRx [N],Tyre x Forces [N].fRLx [N],Tyre x Forces [N].fRRx [N],Tyre y Forces [N].fFLy [N],Tyre y Forces [N].fFRy [N],Tyre y Forces [N].fRLy [N],Tyre y Forces [N].fRRy [N],Tyre My Moments [Nm].mFLy [Nm],Tyre My Moments [Nm].mFRy [Nm],Tyre My Moments [Nm].mRLy [Nm],Tyre My Moments [Nm].mRRy [Nm]
  Lateral Dynamics : Subsystem
  Longitudinal Dynamics : Subsystem
  Pitch Dynamics : Subsystem
  Roll Dynamics : Subsystem
  Steer Input 1 : InportShadow
  Steer Input 2 : InportShadow
  Tyre Forces and Moments 1 : InportShadow  Port=2
  Tyre Forces and Moments 2 : InportShadow  Port=2
  Tyre Forces and Moments 3 : InportShadow  Port=2
  Vertical Dynamics : Subsystem
  Yaw Dynamics : Subsystem
  unsprung masses outputs{1..5} (5 alike) : InportShadow  Port=3
  Sprung mass outputs : Outport
  tag scope: ay=global
  wires:
  Yaw Dynamics/2(psi_dot [rad/s]) -> Bus Creator3/2, [psi_dot]  "psi_dot [rad/s]"
  Lateral Dynamics/2(Vy [m/s]) -> [Vy], Bus Creator2/2  "Vy [m/s]"
  Longitudinal Dynamics/2(Vx [m/s]) -> [Vx], Bus Creator1/2  "Vx [m/s]"
  Longitudinal Dynamics/3(longitudinal x [m]) -> [x], Bus Creator1/3  "x [m]"
  Bus Selector6/2 -> Longitudinal Dynamics/6(fFRx [N])  "<fFRx [N]>"
  Longitudinal Dynamics/1(ax [m/s^2]) -> [ax], Bus Creator1/1  "ax [m/s^2]"
  Yaw Dynamics/1(psi_dot_dot [rad/s^2]) -> Bus Creator3/1, [psi_dot_dot]  "psi_dot_dot [rad/s^2]"
  Yaw Dynamics/3(psi [rad]) -> [psi], Bus Creator3/3  "psi [rad]"
  Bus Selector1/3 -> Vertical Dynamics/3(zRR_dot [m/s])  "<zRR_dot [m/s]>"
  Bus Selector1/1 -> Vertical Dynamics/1(zFL_dot [m/s])  "<zFL_dot [m/s]>"
  Bus Selector1/2 -> Vertical Dynamics/2(ZFR_dot [m/s])  "<zFR_dot [m/s]>"
  Vertical Dynamics/3(vertical z [m]) -> Bus Creator4/3, [z]  "z [m]"
  Roll Dynamics/3(phi [rad]) -> [phi], Bus Creator5/3  "phi [rad]"
  Pitch Dynamics/3(theta [rad]) -> Bus Creator6/3, [theta]  "theta [rad]"
  Vertical Dynamics/2(Vz [m/s]) -> Bus Creator4/2, [Vz]  "Vz [m/s]"
  Vertical Dynamics/1(Vz_dot [m/s^2]) -> Bus Creator4/1, [Vz_dot]  "Vz_dot [m/s^2]"
  Roll Dynamics/2(phi_dot [rad/s]) -> [phi_dot], Bus Creator5/2  "phi_dot [rad/s]"
  Roll Dynamics/1(phi_dot_dot [rad/s^2]) -> [phi_dot_dot], Bus Creator5/1  "phi_dot_dot [rad/s^2]"
  Pitch Dynamics/2(theta_dot [rad/s]) -> Bus Creator6/2, [theta_dot]  "theta_dot [rad/s]"
  Pitch Dynamics/1(theta_dot_dot [rad/s^2]) -> Bus Creator6/1, [theta_dot_dot]  "theta_dot_dot [rad/s^2]"
  [z] -> Pitch Dynamics/7(z [m])
  [z] -> Roll Dynamics/7(z [m])
  [Vz] -> Roll Dynamics/1(Vz[m/s])
  [Vz] -> Pitch Dynamics/1(Vz [m/s])
  [phi_dot] -> Vertical Dynamics/7(phi_dot [rad/s])
  [phi_dot] -> Pitch Dynamics/6(phi_dot [rad/s])
  [phi] -> Pitch Dynamics/12(phi [rad])
  [theta_dot] -> Roll Dynamics/6(theta_dot [rad/s])
  [theta_dot] -> Vertical Dynamics/6(theta_dot [rad/s])
  [theta] -> Roll Dynamics/12(theta [rad])
  [Vz] -> Longitudinal Dynamics/20(Vz [m/s])
  [Vz] -> Lateral Dynamics/20(Vz [m/s])
  [phi_dot] -> Lateral Dynamics/19(phi_dot [rad/s])
  [theta_dot] -> Longitudinal Dynamics/19(theta_dot [rad/s])
  Lateral Dynamics/1(ay [m/s^2]) -> [ay], Bus Creator2/1  "ay [m/s^2]"
  Lateral Dynamics/3(lateral y [m]) -> [y], Bus Creator2/3  "y [m]"
  [theta] -> Vertical Dynamics/13(theta [rad])
  [phi] -> Vertical Dynamics/14(phi [rad])
  Bus Selector/3 -> Vertical Dynamics/11(zRR [m])  "<zRR [m]>"
  Bus Selector/1 -> Vertical Dynamics/9(zFL [m])  "<zFL [m]>"
  Bus Selector/2 -> Vertical Dynamics/10(zFR [m])  "<zFR [m]>"
  Bus Selector/4 -> Vertical Dynamics/12(zRL [m])  "<zRL [m]>"
  Bus Selector1/4 -> Vertical Dynamics/4(zRL_dot [m/s])  "<zRL_dot [m/s]>"
  Bus Selector3/2 -> Roll Dynamics/3(zFR_dot [m/s^2])  "<zFR_dot [m/s]>"
  Bus Selector3/1 -> Roll Dynamics/2(zFL_dot [m/s^2])  "<zFL_dot [m/s]>"
  Bus Selector3/4 -> Roll Dynamics/5(zRL_dot [m/s^2])  "<zRL_dot [m/s]>"
  Bus Selector3/3 -> Roll Dynamics/4(zRR_dot [m/s^2])  "<zRR_dot [m/s]>"
  Tyre Forces and Moments/1 -> Bus Selector6/1
  Bus Selector6/1 -> Longitudinal Dynamics/5(fFLx [N])  "<fFLx [N]>"
  Bus Selector6/3 -> Longitudinal Dynamics/7(fRLx [N])  "<fRLx [N]>"
  Bus Selector6/4 -> Longitudinal Dynamics/8(fRRx [N])  "<fRRx [N]>"
  Bus Selector8/2 -> Lateral Dynamics/6(fFRx [N])  "<fFRx [N]>"
  Bus Selector8/1 -> Lateral Dynamics/5(fFLx [N])  "<fFLx [N]>"
  Tyre Forces and Moments 1/1 -> Bus Selector8/1
  Bus Selector8/3 -> Lateral Dynamics/7(fRLx [N])  "<fRLx [N]>"
  Bus Selector8/4 -> Lateral Dynamics/8(fRRx [N])  "<fRRx [N]>"
  Bus Selector10/4 -> Yaw Dynamics/4(fRRy [N])  "<fRRy [N]>"
  Bus Selector10/3 -> Yaw Dynamics/3(fRLy [N])  "<fRLy [N]>"
  Tyre Forces and Moments 2/1 -> Bus Selector10/1
  Bus Selector10/1 -> Yaw Dynamics/1(fFLy [N])  "<fFLy [N]>"
  Bus Selector10/2 -> Yaw Dynamics/2(fFRy [N])  "<fFRy [N]>"
  [ax] -> Pitch Dynamics/13(ax [m/s^2])
  [Vx] -> Lateral Dynamics/17(Vx [m/s])
  [ay] -> Roll Dynamics/13(ay [m/s^2])
  [Vy] -> Vertical Dynamics/8(Vy [m/s])
  [Vx] -> Vertical Dynamics/5(Vx [m/s])
  [Vy] -> Longitudinal Dynamics/17(Vy [m/s])
  [psi_dot] -> Lateral Dynamics/18(psi_dot [rad/s])
  [psi_dot] -> Longitudinal Dynamics/18(psi_dot [rad/s])
  Bus Creator/1 -> Sprung mass outputs/1
  Steer Input [rad]/1 -> Bus Selector12/1
  Bus Selector12/2 -> Longitudinal Dynamics/2(deltaFR [rad])  "<deltaFR [rad]>"
  Bus Selector12/1 -> Longitudinal Dynamics/1(deltaFL [rad])  "<deltaFL [rad]>"
  Bus Selector12/4 -> Longitudinal Dynamics/4(delta RR [rad])  "<deltaRR [rad]>"
  Bus Selector12/3 -> Longitudinal Dynamics/3(delta RL [rad])  "<deltaRL [rad]>"
  Bus Selector13/2 -> Lateral Dynamics/2(deltaFR [rad])  "<deltaFR [rad]>"
  Bus Selector13/3 -> Lateral Dynamics/3(delta RL [rad])  "<deltaRL [rad]>"
  Bus Selector13/4 -> Lateral Dynamics/4(delta RR [rad])  "<deltaRR [rad]>"
  Steer Input 1/1 -> Bus Selector13/1
  Bus Selector13/1 -> Lateral Dynamics/1(deltaFL [rad])  "<deltaFL [rad]>"
  Bus Selector14/3 -> Yaw Dynamics/11(deltaRL [rad])  "<deltaRL [rad]>"
  Bus Selector14/1 -> Yaw Dynamics/9(deltaFL [rad])  "<deltaFL [rad]>"
  Bus Selector14/4 -> Yaw Dynamics/12(deltaRR [rad])  "<deltaRR [rad]>"
  Bus Selector14/2 -> Yaw Dynamics/10(deltaFR [rad])  "<deltaFR [rad]>"
  Steer Input 2/1 -> Bus Selector14/1
  Bus Creator6/1 -> Bus Creator/6  "Pitch Dynamics"
  Bus Creator5/1 -> Bus Creator/5  "Roll Dynamics"
  Bus Creator4/1 -> Bus Creator/4  "Vertical Dynamics"
  Bus Creator3/1 -> Bus Creator/3  "Yaw dynamics"
  Bus Creator2/1 -> Bus Creator/2  "Lateral Dynamics"
  Bus Creator1/1 -> Bus Creator/1  "Longitudinal Dynamics"
  Bus Selector10/5 -> Yaw Dynamics/5(fFLx [N])  "<fFLx [N]>"
  Bus Selector10/6 -> Yaw Dynamics/6(fFRx [N])  "<fFRx [N]>"
  Bus Selector10/7 -> Yaw Dynamics/7(fRLx [N])  "<fRLx [N]>"
  Bus Selector10/8 -> Yaw Dynamics/8(fRRx [N])  "<fRRx [N]>"
  Bus Selector8/5 -> Lateral Dynamics/9(fFLy [N])  "<fFLy [N]>"
  Bus Selector8/6 -> Lateral Dynamics/10(fFRy [N])  "<fFRy [N]>"
  Bus Selector8/7 -> Lateral Dynamics/11(fRLy [N])  "<fRLy [N]>"
  Bus Selector8/8 -> Lateral Dynamics/12(fRRy [N])  "<fRRy [N]>"
  Bus Selector6/5 -> Longitudinal Dynamics/9(fFLy [N])  "<fFLy [N]>"
  Bus Selector6/6 -> Longitudinal Dynamics/10(fFRy [N])  "<fFRy [N]>"
  Bus Selector6/7 -> Longitudinal Dynamics/11(fRLy [N])  "<fRLy [N]>"
  Bus Selector6/8 -> Longitudinal Dynamics/12(fRRy [N])  "<fRRy [N]>"
  Bus Selector2/3 -> Roll Dynamics/10(zRR [m])  "<zRR [m]>"
  Bus Selector2/4 -> Roll Dynamics/11(zRL [m])  "<zRL [m]>"
  Bus Selector2/1 -> Roll Dynamics/8(zFL [m])  "<zFL [m]>"
  Bus Selector2/2 -> Roll Dynamics/9(zFR [m])  "<zFR [m]>"
  Bus Selector5/3 -> Pitch Dynamics/4(zRR_dot [m/s])  "<zRR_dot [m/s]>"
  Bus Selector5/4 -> Pitch Dynamics/5(zRL_dot [m/s])  "<zRL_dot [m/s]>"
  Bus Selector5/1 -> Pitch Dynamics/2(zFL_dot [m/s])  "<zFL_dot [m/s]>"
  Bus Selector5/2 -> Pitch Dynamics/3(zFR_dot [m/s])  "<zFR_dot [m/s]>"
  Bus Selector4/2 -> Pitch Dynamics/9(zFR [m])  "<zFR [m]>"
  Bus Selector4/1 -> Pitch Dynamics/8(zFL [m])  "<zFL [m]>"
  Bus Selector4/4 -> Pitch Dynamics/11(zRL [m])  "<zRL [m]>"
  Bus Selector4/3 -> Pitch Dynamics/10(zRR [m])  "<zRR [m]>"
  unsprung masses outputs/1 -> Bus Selector1/1
  unsprung masses outputs1/1 -> Bus Selector/1
  unsprung masses outputs2/1 -> Bus Selector3/1
  unsprung masses outputs3/1 -> Bus Selector5/1
  unsprung masses outputs4/1 -> Bus Selector4/1
  unsprung masses outputs5/1 -> Bus Selector2/1
  Tyre Forces and Moments 3/1 -> Bus Selector7/1
  Bus Selector7/1 -> Yaw Dynamics/13(mFLz)  "<mFLz [Nm]>"
  Bus Selector7/2 -> Yaw Dynamics/14(mFRz)  "<mFRz [Nm]>"
  Bus Selector7/3 -> Yaw Dynamics/15(mRLz)  "<mRLz [Nm]>"
  Bus Selector7/4 -> Yaw Dynamics/16(mRRz)  "<mRRz [Nm]>"
  Bus Selector6/9 -> Longitudinal Dynamics/13(mFLy [Nm])  "<mFLy [Nm]>"
  Bus Selector6/10 -> Longitudinal Dynamics/14(mFRy [Nm])  "<mFRy [Nm]>"
  Bus Selector6/11 -> Longitudinal Dynamics/15(mRLy [Nm])  "<mRLy [Nm]>"
  Bus Selector6/12 -> Longitudinal Dynamics/16(mRRy [Nm])  "<mRRy [Nm]>"
  Bus Selector8/9 -> Lateral Dynamics/13(mFLy [Nm])  "<mFLy [Nm]>"
  Bus Selector8/10 -> Lateral Dynamics/14(mFRy [Nm])  "<mFRy [Nm]>"
  Bus Selector8/11 -> Lateral Dynamics/15(mRLy [Nm])  "<mRLy [Nm]>"
  Bus Selector8/12 -> Lateral Dynamics/16(mRRy [Nm])  "<mRRy [Nm]>"
  [Vx] -> Pitch Dynamics/14(Vx [m/s])
  [Vx] -> Roll Dynamics/14(Vx [m/s])

== system VDSE_2018b/14-DOF VEHICLE MODEL/POWERTRAIN AND BRAKES ==
  Wheels speed [rad/s] : Inport
  Driver : Inport  Port=2
  Braking : Subsystem
  Bus Creator : BusCreator  Inputs=4
  Demux : Demux
  Enable Powertrain : Subsystem
  Engine and Gear Box : Subsystem
  Integrator{,1..3} (4 alike) : Integrator
  Overall Torque Calculation : Subsystem
  Torques [Nm] : Outport
  tag scope: angleFL=global, angleFR=global, angleRL=global, angleRR=global, omegaFL=global, omegaFR=global, omegaRL=global, omegaRR=global
  wires:
  Bus Creator/1 -> Torques [Nm]/1
  Driver/1 -> Engine and Gear Box/1(THROTTLE [%]), Braking/1(BRAKING [%])
  Demux/1 -> Engine and Gear Box/2(OMEGA_FL [rad/s]), [omegaFL], Integrator/1  "omegaFL"
  Demux/2 -> Engine and Gear Box/3(OMEGA_FR [rad/s]), [omegaFR], Integrator1/1  "omegaFR"
  Demux/3 -> Engine and Gear Box/4(OMEGA_RL [rad/s]), [omegaRL], Integrator2/1  "omegaRL"
  Demux/4 -> Engine and Gear Box/5(OMEGA_RR [rad/s]), [omegaRR], Integrator3/1  "omegaRR"
  Wheels speed [rad/s]/1 -> Demux/1  "omega [rad/s]"
  Integrator/1 -> [angleFL]
  Integrator1/1 -> [angleFR]
  Integrator2/1 -> [angleRL]
  Integrator3/1 -> [angleRR]
  Engine and Gear Box/1(TENGINE_FL_atWheels [Nm]) -> Overall Torque Calculation/5(TENGINE_FL_atWheels [Nm])
  Engine and Gear Box/2(TENGINE_FR_atWheels [Nm]) -> Overall Torque Calculation/6(TENGINE_FR_atWheels [Nm])
  Engine and Gear Box/3(TENGINE_RL_atWheels [Nm]) -> Overall Torque Calculation/7(TENGINE_RL_atWheels [Nm])
  Engine and Gear Box/4(TENGINE_RR_atWheels [Nm]) -> Overall Torque Calculation/8(TENGINE_RR_atWheels [Nm])
  Overall Torque Calculation/1(TFL [Nm]) -> Enable Powertrain/1(<TFL [Nm]>)
  Overall Torque Calculation/2(TFR [Nm]) -> Enable Powertrain/2(<TFR [Nm]>)
  Overall Torque Calculation/3(TRL [Nm]) -> Enable Powertrain/3(<TRL [Nm]>)
  Overall Torque Calculation/4(TRR [Nm]) -> Enable Powertrain/4(<TRR [Nm]>)
  Enable Powertrain/1(TFL [Nm]) -> Bus Creator/1  "TFL [Nm]"
  Enable Powertrain/2(TFR [Nm]) -> Bus Creator/2  "TFR [Nm]"
  Enable Powertrain/3(TRL [Nm]) -> Bus Creator/3  "TRL [Nm]"
  Enable Powertrain/4(TRR [Nm]) -> Bus Creator/4  "TRR [Nm]"
  Braking/1(TBRAKE_FL_atWheels [Nm]) -> Overall Torque Calculation/1(TBRAKE_FL_atWheels [Nm])
  Braking/2(TBRAKE_FR_atWheels [Nm]) -> Overall Torque Calculation/2(TBRAKE_FR_atWheels [Nm])
  Braking/3(TBRAKE_RL_atWheels [Nm]) -> Overall Torque Calculation/3(TBRAKE_RL_atWheels [Nm])
  Braking/4(TBRAKE_RR_atWheels [Nm]) -> Overall Torque Calculation/4(TBRAKE_RR_atWheels [Nm])

== system VDSE_2018b/14-DOF VEHICLE MODEL/SUSPENSION ==
  note: DYNAMIC LOAD TRANSFER
  note: SUSPENSION
  note: SUSPENSION
  yfront_road [m] : Inport
  yrear_road [m] : Inport  Port=2
  sprung mass outputs : Inport  Port=3
  Bus Creator : BusCreator  Inputs=4
  Bus Creator1 : BusCreator  Inputs=4
  Bus Creator2 : BusCreator  Inputs=4
  Bus Creator3 : BusCreator  Inputs=3
  Bus Selector : BusSelector  OutputSignals=Vertical Dynamics.z [m],Vertical Dynamics.Vz [m/s],Roll Dynamics.phi [rad],Roll Dynamics.phi_dot [rad/s],Pitch Dynamics.theta [rad],Pitch Dynamics.theta_dot [rad/s]
  Bus Selector1 : BusSelector  OutputSignals=Vertical Dynamics.z [m],Vertical Dynamics.Vz [m/s],Roll Dynamics.phi [rad],Roll Dynamics.phi_dot [rad/s],Pitch Dynamics.theta [rad],Pitch Dynamics.theta_dot [rad/s]
  Bus Selector2 : BusSelector  OutputSignals=Longitudinal Dynamics.ax [m/s^2],Lateral Dynamics.ay [m/s^2]
  FRONT SUSPENSION : Subsystem
  Load Transfer : Subsystem
  REAR SUSPENSION : Subsystem
  sprung mass inputs1 : InportShadow  Port=3
  " Unsprung masses output" : Outport
  wires:
  Bus Creator/1 -> Load Transfer/3(Tyre z Forces [N])
  yrear_road [m]/1 -> REAR SUSPENSION/7(yrear_road [m])
  REAR SUSPENSION/2(fRLz [N]) -> [fRLz]  "fRLz [N]"
  yfront_road [m]/1 -> FRONT SUSPENSION/7(yfront_road [m])
  FRONT SUSPENSION/1(fFRz [N]) -> [fFRz]  "fFRz [N]"
  REAR SUSPENSION/1(fRRz [N]) -> [fRRz]  "fRRz [N]"
  Bus Selector/2 -> FRONT SUSPENSION/2(Vz [m/s])  "<Vz [m/s]>"
  [fFLz] -> Bus Creator/1
  [fFRz] -> Bus Creator/2
  [fRLz] -> Bus Creator/3
  [fRRz] -> Bus Creator/4
  [zFL] -> Bus Creator2/1
  [zFR] -> Bus Creator2/2
  [zRL] -> Bus Creator2/3
  [zRR] -> Bus Creator2/4
  [zFL_dot] -> Bus Creator1/1
  [zFR_dot] -> Bus Creator1/2
  [zRL_dot] -> Bus Creator1/3
  [zRR_dot] -> Bus Creator1/4
  FRONT SUSPENSION/2(fFLz [N]) -> [fFLz]  "fFLz [N]"
  FRONT SUSPENSION/5(zFL [m]) -> [zFL]  "zFL [m]"
  FRONT SUSPENSION/3(zFR [m]) -> [zFR]  "zFR [m]"
  FRONT SUSPENSION/4(zFR_dot [m/s]) -> [zFR_dot]  "zFR_dot [m/s]"
  FRONT SUSPENSION/6(zFL_dot [m/s]) -> [zFL_dot]  "zFL_dot [m/s]"
  REAR SUSPENSION/3(zRR [m]) -> [zRR]  "zRR [m]"
  REAR SUSPENSION/4(zRR_dot [m/s]) -> [zRR_dot]  "zRR_dot [m/s]"
  REAR SUSPENSION/5(zRL [m]) -> [zRL]  "zRL [m]"
  REAR SUSPENSION/6(zRL_dot [m/s]) -> [zRL_dot]  "zRL_dot [m/s]"
  Bus Selector/1 -> FRONT SUSPENSION/1(z [m])  "<z [m]>"
  Bus Selector/3 -> FRONT SUSPENSION/3(phi [rad])  "<phi [rad]>"
  Bus Selector/4 -> FRONT SUSPENSION/4(phi_dot [rad/s])  "<phi_dot [rad/s]>"
  Bus Selector/5 -> FRONT SUSPENSION/5(theta [rad])  "<theta [rad]>"
  Bus Selector/6 -> FRONT SUSPENSION/6(theta_dot [rad/s])  "<theta_dot [rad/s]>"
  Bus Selector1/6 -> REAR SUSPENSION/6(theta_dot [rad/s])  "<theta_dot [rad/s]>"
  Bus Selector1/4 -> REAR SUSPENSION/4(phi_dot [rad/s])  "<phi_dot [rad/s]>"
  sprung mass outputs/1 -> Bus Selector1/1, Bus Selector/1
  Bus Selector1/5 -> REAR SUSPENSION/5(theta [rad])  "<theta [rad]>"
  Bus Selector1/1 -> REAR SUSPENSION/1(z [m])  "<z [m]>"
  Bus Selector1/2 -> REAR SUSPENSION/2(Vz [m/s])  "<Vz [m/s]>"
  Bus Selector1/3 -> REAR SUSPENSION/3(phi [rad])  "<phi [rad]>"
  Load Transfer/1(Tyres z forces [N]) -> Bus Creator3/1  "Unsprung masses z Forces [N]"
  sprung mass inputs1/1 -> Bus Selector2/1
  Bus Selector2/1 -> Load Transfer/1(ax [m/s^2])  "<ax [m/s^2]>"
  Bus Selector2/2 -> Load Transfer/2(ay [m/s^2])  "<ay [m/s^2]>"
  Bus Creator2/1 -> Bus Creator3/2  "Unsprung masses z displacement [m]"
  Bus Creator3/1 -> " Unsprung masses output"/1
  Bus Creator1/1 -> Bus Creator3/3  "Unsprung masses z Velocities [m/s]"

== system VDSE_2018b/14-DOF VEHICLE MODEL/WHEEL ASSEMBLY ==
  note: 1) Add Subsystem or Model blocks as valid variant choices.
      | 2) You cannot connect blocks at this level. At simulation, connectivity is automatically
      | determined, based on the active variant and port name matching.
  steer input [rad] : Inport
  sprung mass outputs : Inport  Port=2
  unsprung masses outputs : Inport  Port=3
  Torques [Nm] : Inport  Port=4
  WHEEL ASSEMBLY BCD : Subsystem  VariantControl=WHEEL_ASSEMBLY_BCD
  WHEEL ASSEMBLY MFEVAL : Subsystem  VariantControl=WHEEL_ASSEMBLY_MFEVAL
  WHEEL ASSEMBLY PACEIJKA : Subsystem  VariantControl=WHEEL_ASSEMBLY_PACEIJKA
  Tyre Forces and Moments : Outport
  Wheel Speeds [rad/s] : Outport  Port=2

== system VDSE_2018b/RESULTS/Subsystem2 ==
  vx : Inport
  vy : Inport  Port=2
  psi : Inport  Port=3
  Add : Sum  Inputs=+-
  Add1 : Sum
  Cos : Trigonometry  Operator=cos
  Cos1 : Trigonometry
  Cos2 : Trigonometry  Operator=cos
  Cos3 : Trigonometry
  Product{,1..3} (4 alike) : Product
  vx_inertialFrame : Outport
  vy_inertialFrame : Outport  Port=2
  wires:
  Cos1/1 -> Product1/1
  Add/1 -> vx_inertialFrame/1
  Product1/1 -> Add/2
  Product/1 -> Add/1
  Cos/1 -> Product/2
  vx/1 -> Product3/2, Product/1
  Cos2/1 -> Product2/2
  Product2/1 -> Add1/1
  Product3/1 -> Add1/2
  Cos3/1 -> Product3/1
  vy/1 -> Product2/1, Product1/2
  psi/1 -> Cos/1, Cos1/1, Cos2/1, Cos3/1
  Add1/1 -> vy_inertialFrame/1
